simulink model "uz_pos_to_speed_pll"  (R2023a)
settings: Solver=FixedStepDiscrete  StartTime=0.0  StopTime=5*100e-6  RelTol=1e-3  EnableMultiTasking=on
PreLoadFcn:
  | uz_setCodegenPaths
model workspace (MATLAB code in the model file):
  | cmdLim = Simulink.Parameter;
  | cmdLim.Value = 15;
  | cmdLim.Description = 'Limit for controlling the maximum surface command angle.';
  | cmdLim.Min = 0;
  | cmdLim.Max = 90;
  | cmdLim.DocUnits = 'deg';
  | 
  | dispGain = Simulink.Parameter;
  | dispGain.Value = 0.75;
  | dispGain.Description = 'Gain applied to the displacement error.';
  | dispGain.Min = 0;
  | dispGain.Max = [];
  | dispGain.DocUnits = 'deg/sec/deg';
  | 
  | dispLim = Simulink.Parameter;
  | dispLim.Value = 30;
  | dispLim.Description = 'Limit for controlling the maximum commanded angle.';
  | dispLim.Min = 0;
  | dispLim.Max = 180;
  | dispLim.DocUnits = 'deg';
  | 
  | intGain = Simulink.Parameter;
  | intGain.Value = 0.5;
  | intGain.Description = 'Gain applied to the integral error.';
  | intGain.Min = 0;
  | intGain.Max = [];
  | intGain.DocUnits = 'deg/sec/deg/sec';
  | 
  | intLim = Simulink.Parameter;
  | intLim.Value = 5;
  | intLim.Description = 'Limit for controlling the maximum commanded angle.';
  | intLim.Min = 0;
  | intLim.Max = 90;
  | intLim.DocUnits = 'deg';
  | 
  | rateGain = Simulink.Parameter;
  | rateGain.Value = 2;
  | rateGain.Description = 'Gain applied to the rate error.';
  | rateGain.Min = 0;
  | rateGain.Max = [];
  | rateGain.DocUnits = 'deg/deg/sec';
  | 
  | rateLim = Simulink.Parameter;
  | rateLim.Value = 6;
  | rateLim.Description = 'Limit for controlling the maximum commanded angle.';
  | rateLim.Min = 0;
  | rateLim.Max = 180;
  | rateLim.DocUnits = 'deg/sec';
  | 
  | hdgGain = Simulink.Parameter;
  | hdgGain.Value = 0.015;
undefined symbols (not defined in the file or in its folder): motor, PLL
libraries: simulink x1
settings Model: RequirementInfo={} %GIDa_fe9045fd_0412_4b6e_8206_617cc20e6fde  Creator=ts  LastModifiedBy=micha
settings SolverCC: AlgebraicLoopSolver=TrustRegion  PositivePriorityOrder=on  AutoInsertRateTranBlk=on
settings DataIOCC: SaveOutput=off  SignalLogging=off  DSMLogging=off  SaveTime=off
settings OptimizationCC: DefaultParameterBehavior=Inlined  UseDivisionForNetSlopeComputation=on  GainParamInheritBuiltInType=on  UseFloatMulNetSlope=on  UseSpecifiedMinMax=on  InlineInvariantSignals=on  PassReuseOutputArgsAs=Individual arguments  ZeroExternalMemoryAtStartup=off  ZeroInternalMemoryAtStartup=off  NoFixptDivByZeroProtection=on  EfficientFloat2IntCast=on  LifeSpan=1  MaxStackSize=64  OptimizeBlockOrder=speed  DifferentSizesBufferReuse=on  EfficientTunableParamExpr=on
settings DebuggingCC: UnconnectedInputMsg=warning  UnconnectedOutputMsg=warning  UnconnectedLineMsg=warning  AllowSymbolicDim=off  SFUnexpectedBacktrackingDiag=warning  SFNoUnconditionalDefaultTransitionDiag=warning  SFExecutionAtInitializationDiag=none  ArithmeticOperatorsInVariantConditions=warning
settings HardwareCC: ProdBitPerPointer=32  ProdBitPerSizeT=32  ProdBitPerPtrDiffT=32  ProdLargestAtomicInteger=Long  ProdLargestAtomicFloat=Double  ProdWordSize=32  ProdLongLongMode=on  ProdHWDeviceType=ARM Compatible->ARM Cortex-R  HardwareBoardFeatureSet=SoCBlockset
settings ModelReferenceCC: EnableRefExpFcnMdlSchedulingChecks=on
settings SFSimCC: MATLABDynamicMemAlloc=off
settings RTWCC: Description=Embedded Coder  SystemTargetFile=ert.tlc  GenCodeOnly=on  TemplateMakefile=ert_default_tmf  GenerateReport=on  BuildConfiguration=Faster Runs  IncludeHyperlinkInReport=on  LaunchReport=on  GenerateTraceInfo=on  GenerateTraceReport=on  GenerateTraceReportSl=on  GenerateTraceReportSf=on  GenerateTraceReportEml=on  GenerateCodeMetricsReport=on  CheckMdlBeforeBuild=Warning  DLArmComputeVersion=19.05
settings CodeAppCC: ForceParamTrailComments=on  IgnoreCustomStorageClasses=off  OperatorAnnotations=on  SimulinkDataObjDesc=on  SFDataObjDesc=on  MATLABFcnDesc=on  CustomSymbolStrGlobalVar=rt$N$M  CustomSymbolStrType=$N$M  CustomSymbolStrFcn=$N$M$F  CustomSymbolStrMacro=$N$M  InsertBlockDesc=on  StateflowObjectComments=on  MATLABSourceComments=on  EnableCustomComments=on  ReqsInCode=on
settings ERTTargetCC: TargetLangStandard=C99 (ISO)  CodeReplacementLibrary=GNU C99 extensions  MultiwordLength=2048  IncludeMdlTerminateFcn=off  CombineSignalStateStructs=on  SuppressErrorStatus=on  IncludeFileDelimiter=UseQuote  SupportAbsoluteTime=off  CodeInterfacePackaging=Reusable function  SupportNonFinite=off  RemoveResetFunc=off  InlinedParameterPlacement=NonHierarchical  MultiInstanceErrorCode=Warning  RootIOFormat=Part of model data structure  ERTCustomFileTemplate=example_file_process.tlc  GlobalDataDefinition=InSourceFile  GlobalDataReference=InSourceFile  ERTFilePackagingFormat=CompactWithDataFile
settings ConfigComp: CovScope=ReferencedModels  CovSaveName=covdata_rollAP  CovMetricSettings=dcmtrwe  CovHTMLOptions=-sRT=1 -aTS=1 -bRG=1 -bTC=1 -hTR=1 -nFC=0 -scm=1 -bcm=1 -xEv=0  CovSaveCumulativeToWorkspaceVar=on  CovSaveSingleToWorkspaceVar=on  CovCumulativeVarName=covCumulativeData_rollAP  CovReportOnPause=off  CovExternalEMLEnable=off  CovSFcnEnable=off

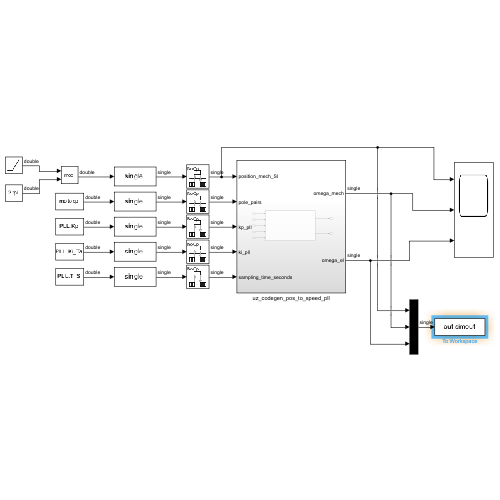
[thumbnail: Simulink's stored preview of the top-level diagram]
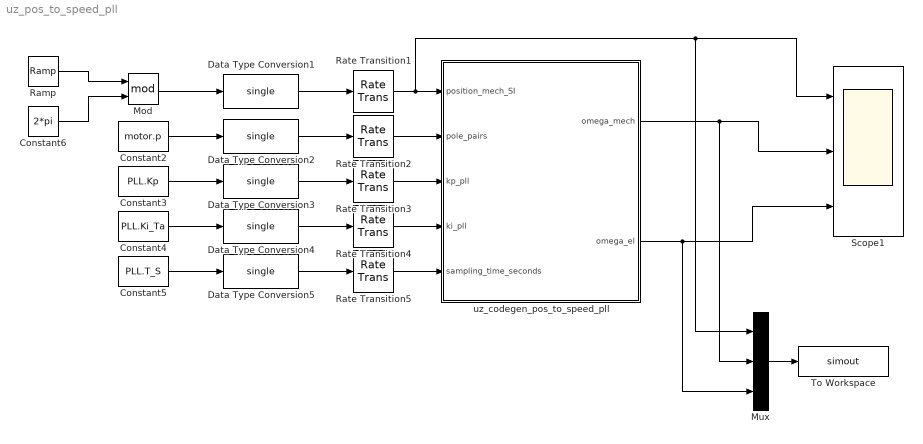
== system uz_pos_to_speed_pll ==
  Constant2 : Constant  Value=motor.p  SampleTime=-1
  Constant3 : Constant  Value=PLL.Kp  SampleTime=-1
  Constant4 : Constant  Value=PLL.Ki_Ta  SampleTime=-1
  Constant5 : Constant  Value=PLL.T_S  SampleTime=-1
  Constant6 : Constant  Value=2*pi  SampleTime=-1
  Data Type Conversion{1..5} (5 alike) : DataTypeConversion  OutDataTypeStr=single  SaturateOnIntegerOverflow=off  RndMeth=Floor
  Mod : Math  Operator=mod
  Mux : Mux  Inputs=3
  Ramp : simulink/Sources/Ramp  slope=2*pi*50  start=0  InitialOutput=0
  Rate Transition{1..5} (5 alike) : RateTransition  OutPortSampleTime=PLL.T_S
  Scope1 : Scope  NumInputPorts=3
  To Workspace : ToWorkspace  VariableName=simout  SaveFormat=Timeseries  SampleTime=100e-6
  uz_codegen_pos_to_speed_pll : Subsystem
  wires:
  Data Type Conversion1/1 -> Rate Transition1/1
  Data Type Conversion2/1 -> Rate Transition2/1
  Data Type Conversion3/1 -> Rate Transition3/1
  Data Type Conversion4/1 -> Rate Transition4/1
  Data Type Conversion5/1 -> Rate Transition5/1
  Rate Transition1/1 -> Mux/1, Scope1/1, uz_codegen_pos_to_speed_pll/1(position_mech_SI)
  Rate Transition2/1 -> uz_codegen_pos_to_speed_pll/2(pole_pairs)
  Rate Transition4/1 -> uz_codegen_pos_to_speed_pll/4(ki_pll)
  Rate Transition3/1 -> uz_codegen_pos_to_speed_pll/3(kp_pll)
  Rate Transition5/1 -> uz_codegen_pos_to_speed_pll/5(sampling_time_seconds)
  Constant2/1 -> Data Type Conversion2/1
  Constant3/1 -> Data Type Conversion3/1
  Constant4/1 -> Data Type Conversion4/1
  Constant5/1 -> Data Type Conversion5/1
  Ramp/1 -> Mod/1
  Mod/1 -> Data Type Conversion1/1
  Constant6/1 -> Mod/2
  uz_codegen_pos_to_speed_pll/2(omega_el) -> Mux/3, Scope1/3
  Mux/1 -> To Workspace/1
  uz_codegen_pos_to_speed_pll/1(omega_mech) -> Mux/2, Scope1/2

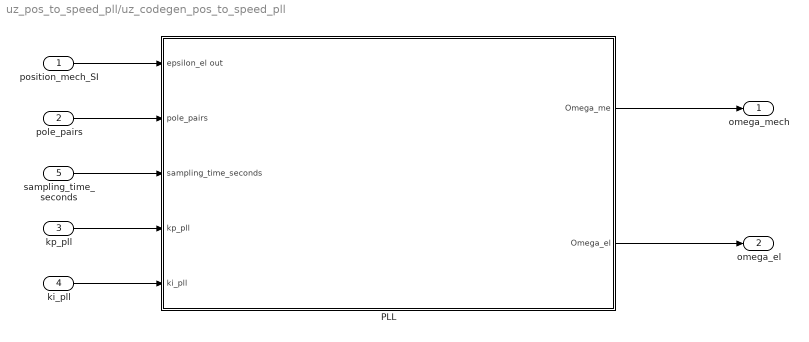
== system uz_pos_to_speed_pll/uz_codegen_pos_to_speed_pll ==
  position_mech_SI : Inport
  pole_pairs : Inport  Port=2
  kp_pll : Inport  Port=3
  ki_pll : Inport  Port=4
  sampling_time_seconds : Inport  Port=5
  PLL : Subsystem
  omega_mech : Outport
  omega_el : Outport  Port=2
  wires:
  position_mech_SI/1 -> PLL/1(epsilon_el out)
  pole_pairs/1 -> PLL/2(pole_pairs)
  kp_pll/1 -> PLL/4(kp_pll)
  ki_pll/1 -> PLL/5(ki_pll)
  sampling_time_seconds/1 -> PLL/3(sampling_time_seconds)
  PLL/1(Omega_me) -> omega_mech/1
  PLL/2(Omega_el) -> omega_el/1

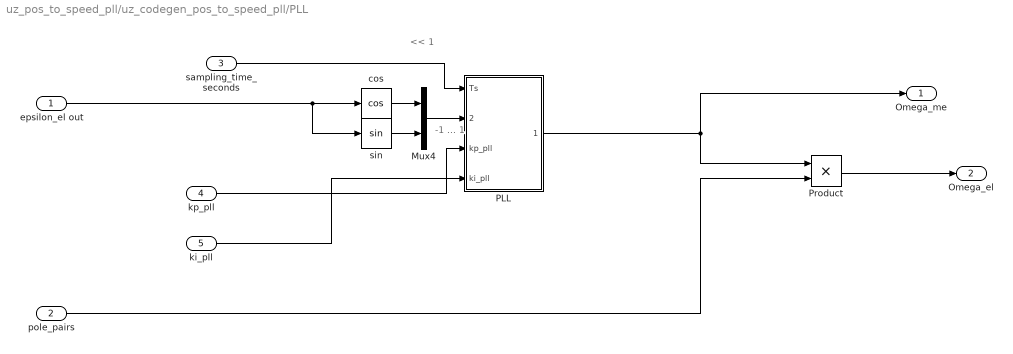
== system uz_pos_to_speed_pll/uz_codegen_pos_to_speed_pll/PLL ==
  note: -1 ... 1
  note: << 1
  epsilon_el out : Inport
  pole_pairs : Inport  Port=2
  sampling_time_seconds : Inport  Port=3
  kp_pll : Inport  Port=4
  ki_pll : Inport  Port=5
  Mux4 : Mux  Inputs=2
  PLL : Subsystem
  Product : Product
  cos : Trigonometry  Operator=cos
  sin : Trigonometry
  Omega_me : Outport
  Omega_el : Outport  Port=2
  wires:
  Mux4/1 -> PLL/2(phi_el_cs)
  sampling_time_seconds/1 -> PLL/1(Ts)
  PLL/1(Omega_mech) -> Omega_me/1, Product/1
  epsilon_el out/1 -> sin/1, cos/1
  sin/1 -> Mux4/2
  cos/1 -> Mux4/1
  pole_pairs/1 -> Product/2
  Product/1 -> Omega_el/1
  kp_pll/1 -> PLL/3(kp_pll)
  ki_pll/1 -> PLL/4(ki_pll)

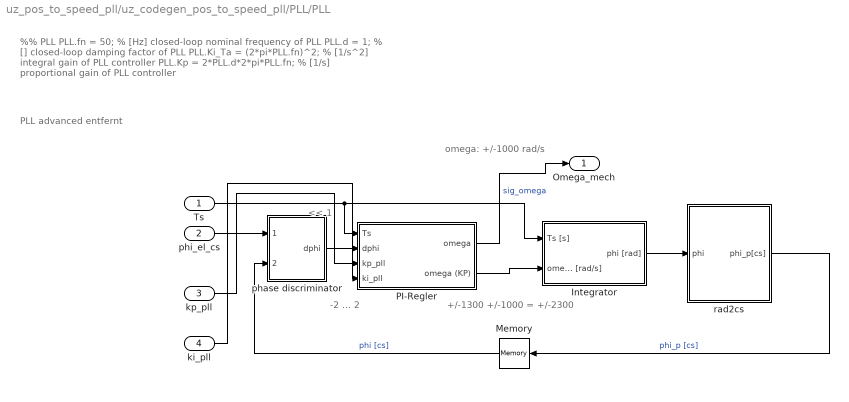
== system uz_pos_to_speed_pll/uz_codegen_pos_to_speed_pll/PLL/PLL ==
  note: %% PLL
      | PLL.fn  =  50;           % [Hz] closed-loop nominal frequency of PLL
      | PLL.d   =  1;            % [] closed-loop damping factor of PLL
      | PLL.Ki_Ta = (2*pi*PLL.fn)^2;    % [1/s^2] integral gain of PLL controller
      | PLL.Kp = 2*PLL.d*2*pi*PLL.fn;   % [1/s] proportional gain of PLL controller
  note: PLL advanced entfernt
  note: -2 ... 2
  note: << 1
  note: +/-1300 +/-1000 = +/-2300
  note: omega: +/-1000 rad/s
  Ts : Inport
  phi_el_cs : Inport  Port=2
  kp_pll : Inport  Port=3
  ki_pll : Inport  Port=4
  Integrator : Subsystem
  Memory : Memory  InitialCondition=[1 0]  InheritSampleTime=on  LinearizeAsDelay=on
  PI-Regler : Subsystem
  phase discriminator : Subsystem
  rad2cs : Subsystem
  Omega_mech : Outport
  wires:
  Ts/1 -> PI-Regler/1(Ts), Integrator/1(Ts [s])
  rad2cs/1(phi_p[cs]) -> Memory/1  "phi_p [cs]"
  phase discriminator/1(dphi) -> PI-Regler/2(dphi)
  Integrator/1(phi [rad]) -> rad2cs/1(phi)
  PI-Regler/2(omega (KP)) -> Integrator/2(omega [rad/s])
  PI-Regler/1(omega) -> Omega_mech/1  "sig_omega"
  phi_el_cs/1 -> phase discriminator/1(phi_x[cs])
  Memory/1 -> phase discriminator/2(phi_e[cs])  "phi [cs]"
  kp_pll/1 -> PI-Regler/3(kp_pll)
  ki_pll/1 -> PI-Regler/4(ki_pll)

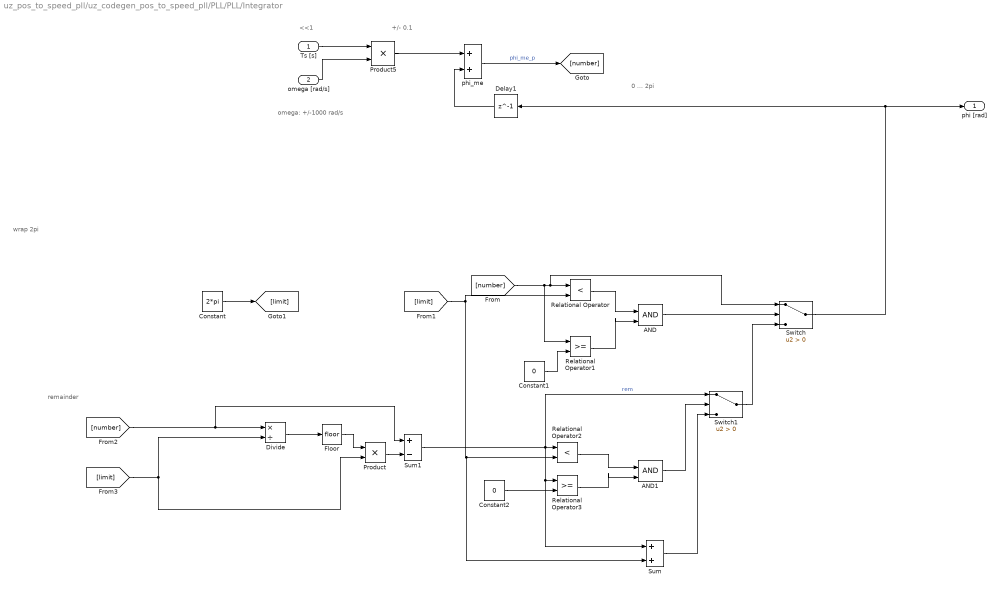
== system uz_pos_to_speed_pll/uz_codegen_pos_to_speed_pll/PLL/PLL/Integrator ==
  note: wrap 2pi
  note: remainder
  note: <<1
  note: omega: +/-1000 rad/s
  note: +/- 0.1
  note: 0 ... 2pi
  Ts [s] : Inport
  omega [rad/s] : Inport  Port=2
  AND : Logic  IconShape=distinctive  AllPortsSameDT=off  OutDataTypeStr=boolean
  AND1 : Logic  IconShape=distinctive  AllPortsSameDT=off  OutDataTypeStr=boolean
  Constant : Constant  Value=2*pi  OutDataTypeStr=single  SampleTime=PLL.T_S
  Constant1 : Constant  Value=0  SampleTime=PLL.T_S
  Constant2 : Constant  Value=0  SampleTime=PLL.T_S
  Delay1 : Delay  DelayLength=1
  Divide : Product  Inputs=*/
  Floor : Rounding
  Product : Product
  Product5 : Product  Inputs=**  InputSameDT=on  RndMeth=Zero  SaturateOnIntegerOverflow=on  OutDataTypeStr=Inherit: Same as first input
  Relational Operator : RelationalOperator  Operator=<  OutDataTypeStr=boolean  RndMeth=Simplest  InputSameDT=off
  Relational Operator1 : RelationalOperator  OutDataTypeStr=boolean  RndMeth=Simplest  InputSameDT=off
  Relational Operator2 : RelationalOperator  Operator=<  OutDataTypeStr=boolean  RndMeth=Simplest  InputSameDT=off
  Relational Operator3 : RelationalOperator  OutDataTypeStr=boolean  RndMeth=Simplest  InputSameDT=off
  Sum : Sum
  Sum1 : Sum  Inputs=+-
  Switch : Switch  Criteria=u2 > Threshold  SaturateOnIntegerOverflow=off  InputSameDT=off
  Switch1 : Switch  Criteria=u2 > Threshold  SaturateOnIntegerOverflow=off  InputSameDT=off
  phi_me : Sum  InputSameDT=on  SaturateOnIntegerOverflow=on  OutDataTypeStr=Inherit: Same as first input
  phi [rad] : Outport
  wires:
  phi_me/1 -> [number]  "phi_me_p"
  Delay1/1 -> phi_me/2
  Ts [s]/1 -> Product5/1
  omega [rad/s]/1 -> Product5/2
  [number] -> Switch/1, Relational Operator/1, Relational Operator1/1
  [limit] -> Sum/2, Relational Operator2/2, Relational Operator/2
  Relational Operator/1 -> AND/1
  Constant1/1 -> Relational Operator1/2
  Relational Operator1/1 -> AND/2
  AND/1 -> Switch/2
  Switch1/1 -> Switch/3
  Relational Operator2/1 -> AND1/1
  Sum1/1 -> Switch1/1, Sum/1, Relational Operator3/1, Relational Operator2/1  "rem"
  Constant2/1 -> Relational Operator3/2
  Relational Operator3/1 -> AND1/2
  AND1/1 -> Switch1/2
  Sum/1 -> Switch1/3
  [limit] -> Divide/2, Product/2
  Divide/1 -> Floor/1
  Floor/1 -> Product/1
  Product/1 -> Sum1/2
  [number] -> Sum1/1, Divide/1
  Product5/1 -> phi_me/1
  Constant/1 -> [limit]
  Switch/1 -> phi [rad]/1, Delay1/1

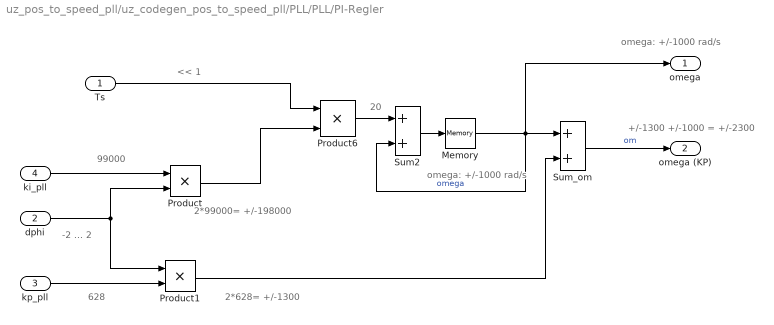
== system uz_pos_to_speed_pll/uz_codegen_pos_to_speed_pll/PLL/PLL/PI-Regler ==
  note: 628
  note: -2 ... 2
  note: 20
  note: 99000
  note: 2*628= +/-1300
  note: 2*99000= +/-198000
  note: << 1
  note: omega: +/-1000 rad/s
  note: +/-1300 +/-1000 = +/-2300
  note: omega: +/-1000 rad/s
  Ts : Inport
  dphi : Inport  Port=2
  kp_pll : Inport  Port=3
  ki_pll : Inport  Port=4
  Memory : Memory  InheritSampleTime=on  LinearizeAsDelay=on
  Product : Product
  Product1 : Product
  Product6 : Product  Inputs=**  InputSameDT=on  RndMeth=Zero  SaturateOnIntegerOverflow=on  OutDataTypeStr=Inherit: Same as first input
  Sum2 : Sum  InputSameDT=on  SaturateOnIntegerOverflow=on  OutDataTypeStr=Inherit: Same as first input
  Sum_om : Sum  InputSameDT=on  SaturateOnIntegerOverflow=on  OutDataTypeStr=Inherit: Same as first input
  omega : Outport
  omega (KP) : Outport  Port=2
  wires:
  Product6/1 -> Sum2/1
  dphi/1 -> Product1/1, Product/2
  Product/1 -> Product6/2
  Sum2/1 -> Memory/1
  Memory/1 -> Sum_om/1, omega/1, Sum2/2  "omega"
  Product1/1 -> Sum_om/2
  Sum_om/1 -> omega (KP)/1  "om"
  Ts/1 -> Product6/1
  ki_pll/1 -> Product/1
  kp_pll/1 -> Product1/2

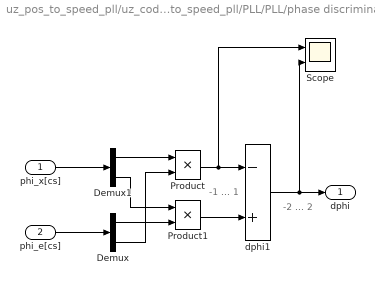
== system uz_pos_to_speed_pll/uz_codegen_pos_to_speed_pll/PLL/PLL/phase discriminator ==
  note: -1 ... 1
  note: -2 ... 2
  phi_x[cs] : Inport  PortDimensions=2
  phi_e[cs] : Inport  Port=2  PortDimensions=2
  Demux : Demux  Outputs=2
      settings: DisplayOption=none
  Demux1 : Demux  Outputs=2
      settings: DisplayOption=none
  Product : Product  Inputs=**  InputSameDT=on  RndMeth=Zero  SaturateOnIntegerOverflow=on  OutDataTypeStr=Inherit: Same as first input
  Product1 : Product  Inputs=**  InputSameDT=on  RndMeth=Zero  SaturateOnIntegerOverflow=on  OutDataTypeStr=Inherit: Same as first input
  Scope : Scope  NumInputPorts=2
  dphi1 : Sum  Inputs=-+  InputSameDT=on  SaturateOnIntegerOverflow=on  OutDataTypeStr=Inherit: Same as first input
  dphi : Outport
  wires:
  dphi1/1 -> Scope/2, dphi/1
  phi_e[cs]/1 -> Demux/1
  Demux1/2 -> Product1/1
  Demux/1 -> Product1/2
  Demux/2 -> Product/2
  Demux1/1 -> Product/1
  Product1/1 -> dphi1/2
  Product/1 -> Scope/1, dphi1/1
  phi_x[cs]/1 -> Demux1/1

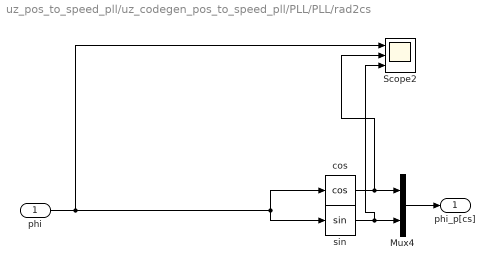
== system uz_pos_to_speed_pll/uz_codegen_pos_to_speed_pll/PLL/PLL/rad2cs ==
  phi : Inport  PortDimensions=1
  Mux4 : Mux  Inputs=2
  Scope2 : Scope  NumInputPorts=3
  cos : Trigonometry  Operator=cos
  sin : Trigonometry
  phi_p[cs] : Outport
  wires:
  phi/1 -> cos/1, sin/1, Scope2/1
  cos/1 -> Scope2/2, Mux4/1
  sin/1 -> Scope2/3, Mux4/2
  Mux4/1 -> phi_p[cs]/1
